simulink model "PIDTu4_2930"  (Simulink 5.0)
settings: Solver=ode4  StartTime=0.0  StopTime=10  FixedStep=0.001  RelTol=1e-3
libraries: simulink_extras x3
settings Model: LastModifiedBy=ThinkPad

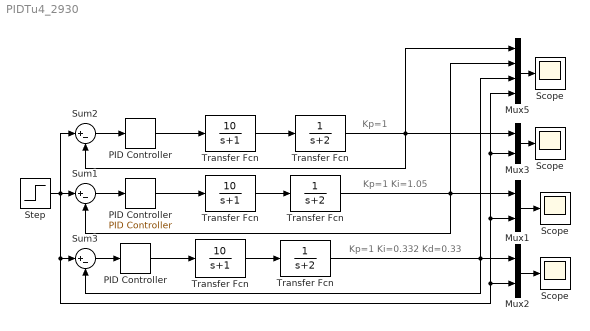
== system PIDTu4_2930 ==
  note: Kp=1
  note: Kp=1 Ki=1.05
  note: Kp=1 Ki=0.332 Kd=0.33
  " PID Controller " : simulink_extras/Additional Linear/PID Controller  P=1  I=1.05  D=0
  " Scope " : Scope
      settings: YMin=-3.5  YMax=1  MaxDataPoints=500000
  " Transfer Fcn" : TransferFcn  Numerator=[10]  Denominator=[1 1]
  " Transfer Fcn  " : TransferFcn  Denominator=[1 2]
  Mux1 : Mux  Inputs=2
  Mux2 : Mux  Inputs=2
  Mux3 : Mux  Inputs=2
  Mux5 : Mux
  PID Controller : simulink_extras/Additional Linear/PID Controller  P=1  I=0.332  D=0.33
  "PID Controller " : simulink_extras/Additional Linear/PID Controller  P=1  I=0  D=0
  Scope : Scope
      settings: YMin=-3.5  YMax=1  MaxDataPoints=500000
  "Scope " : Scope
      settings: YMin=-3.5  YMax=1  SaveName=PIDtu4_30  DataFormat=Array  MaxDataPoints=500000
  "Scope  " : Scope
      settings: YMin=-3.5  YMax=1  SaveName=ScopeData2  MaxDataPoints=500000
  Step : Step  Time=0  SampleTime=0
  Sum1 : Sum  Inputs=|+-  SaturateOnIntegerOverflow=on
  Sum2 : Sum  Inputs=|+-  SaturateOnIntegerOverflow=on
  Sum3 : Sum  Inputs=|+-  SaturateOnIntegerOverflow=on
  "Transfer Fcn " : TransferFcn  Numerator=[10]  Denominator=[1 1]
  "Transfer Fcn    " : TransferFcn  Denominator=[1 2]
  "Transfer Fcn  " : TransferFcn  Denominator=[1 2]
  "Transfer Fcn   " : TransferFcn  Numerator=[10]  Denominator=[1 1]
  wires:
  Mux2/1 -> "Scope  "/1
  "Transfer Fcn  "/1 -> Mux2/1, Sum3/2, Mux5/3
  Step/1 -> Sum1/1, Sum2/1, Sum3/1, Mux2/2, Mux1/2, Mux5/4, Mux3/2
  Mux1/1 -> " Scope "/1
  " Transfer Fcn  "/1 -> Mux5/2, Mux1/1, Sum1/2
  Mux3/1 -> Scope/1
  "PID Controller "/1 -> "Transfer Fcn "/1
  "Transfer Fcn    "/1 -> Mux3/1, Mux5/1, Sum2/2
  Mux5/1 -> "Scope "/1
  Sum2/1 -> "PID Controller "/1
  " PID Controller "/1 -> "Transfer Fcn   "/1
  Sum1/1 -> " PID Controller "/1
  PID Controller/1 -> " Transfer Fcn"/1
  Sum3/1 -> PID Controller/1
  "Transfer Fcn "/1 -> "Transfer Fcn    "/1
  "Transfer Fcn   "/1 -> " Transfer Fcn  "/1
  " Transfer Fcn"/1 -> "Transfer Fcn  "/1
